simulink model "SuperMileage_BMS_Simulink_Model"  (R2023b)
settings: Solver=FixedStepAuto  StartTime=0.0  StopTime=Tspan(end)  FixedStep=Delta_t  RelTol=1e-3
values from neighbouring files (symbols this model uses):
  C = 300    [SuperMileage_BMS.m]
  Q = 4.0*4    (= 16)    [SuperMileage_BMS.m]
  R1 = 0.01    [SuperMileage_BMS.m]
  Rs = 0.01    [SuperMileage_BMS.m]
  SOC_0 = 1.0    (= 1)    [SuperMileage_BMS.m]
settings Model: Creator=leiph  LastModifiedBy=leiph
settings DataIOCC: SaveFormat=StructureWithTime  SaveState=on  TimeSaveName=tout_2C
settings DebuggingCC: UnconnectedInputMsg=warning  UnconnectedOutputMsg=warning  UnconnectedLineMsg=warning
settings ModelReferenceCC: EnableRefExpFcnMdlSchedulingChecks=on
settings RTWCC: DLArmComputeVersion=19.05

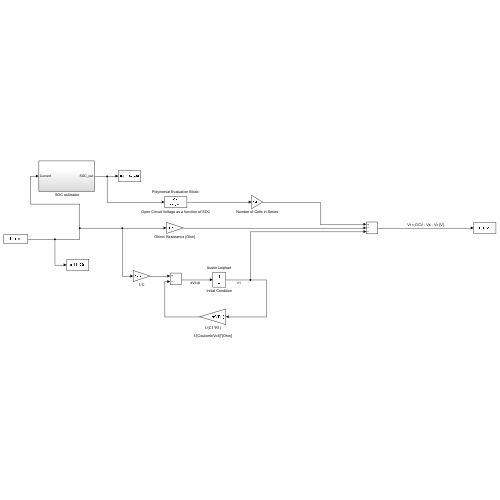
[thumbnail: Simulink's stored preview of the top-level diagram]
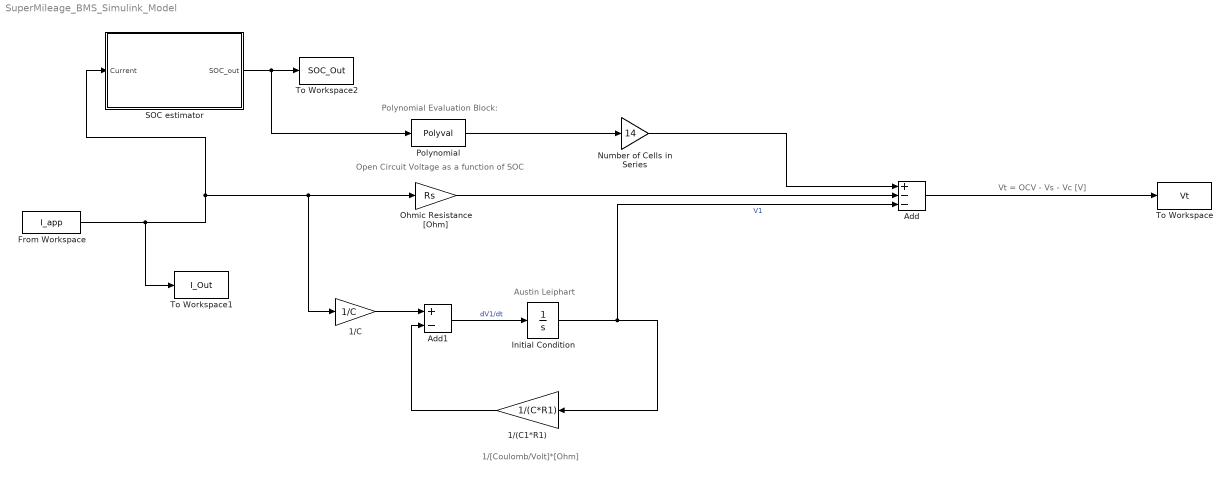
== system SuperMileage_BMS_Simulink_Model ==
  note: 1/[Coulomb/Volt]*[Ohm]
  note: Polynomial Evaluation Block:
  note: Vt = OCV - Vs - Vc [V]
  note: Open Circuit Voltage as a function of SOC
  note: Austin Leiphart
  " SOC estimator" : Subsystem
  1/(C1*R1) : Gain  Gain=1/(C*R1)
  1/C : Gain  Gain=1/C
  Add : Sum  Inputs=+--
  Add1 : Sum  Inputs=+-
  From Workspace : FromWorkspace  VariableName=I_app
  Initial Condition : Integrator
  Number of Cells in Series : Gain  Gain=14
  Ohmic Resistance [Ohm] : Gain  Gain=Rs
  Polynomial : Polyval  Coefs=[1.6155, -3.3842, 3.1980, 2.7675]
  To Workspace : ToWorkspace  VariableName=Vt  SampleTime=-1
      settings: Save2DSignal=2-D array (concatenate along first dimension)
  To Workspace1 : ToWorkspace  VariableName=I_Out  SampleTime=-1
      settings: Save2DSignal=2-D array (concatenate along first dimension)
  To Workspace2 : ToWorkspace  VariableName=SOC_Out  SampleTime=-1
      settings: Save2DSignal=2-D array (concatenate along first dimension)
  wires:
  " SOC estimator"/1(SOC_out) -> Polynomial/1, To Workspace2/1
  Add/1 -> To Workspace/1
  Initial Condition/1 -> 1/(C1*R1)/1, Add/3  "V1"
  Ohmic Resistance [Ohm]/1 -> Add/2
  1/(C1*R1)/1 -> Add1/2
  1/C/1 -> Add1/1
  Add1/1 -> Initial Condition/1  "dV1/dt"
  From Workspace/1 -> To Workspace1/1, 1/C/1, Ohmic Resistance [Ohm]/1, " SOC estimator"/1(Current)
  Polynomial/1 -> Number of Cells in Series/1
  Number of Cells in Series/1 -> Add/1

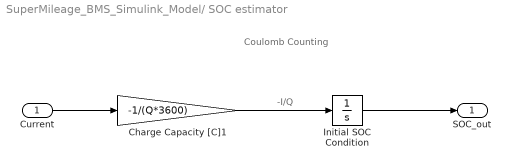
== system SuperMileage_BMS_Simulink_Model/ SOC estimator ==
  note: Coulomb Counting
  note: -I/Q
  Current : Inport
  Charge Capacity [C]1 : Gain  Gain=-1/(Q*3600)
  Initial SOC Condition : Integrator  InitialCondition=SOC_0
  SOC_out : Outport  VectorParamsAs1DForOutWhenUnconnected=off
  wires:
  Charge Capacity [C]1/1 -> Initial SOC Condition/1
  Initial SOC Condition/1 -> SOC_out/1
  Current/1 -> Charge Capacity [C]1/1
